simulink model "STChavelsan"  (R2015b)
settings: Solver=VariableStepAuto  StartTime=0.0  StopTime=10.0  RelTol=1e-3
settings Model: Creator=hyarkin  LastModifiedBy=hyarkin

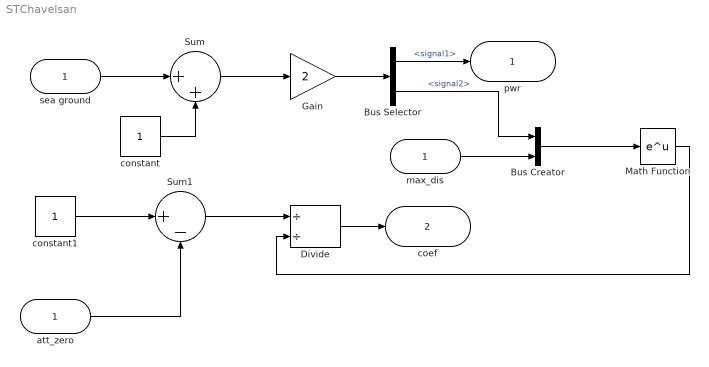
== system STChavelsan ==
  sea ground : Inport
  Bus Creator : BusCreator  Inputs=2
  Bus Selector : BusSelector  OutputSignals=signal1,signal2
  Divide : Product  Inputs=//
  Gain : Gain  Gain=2
  Math Function : Math  SaturateOnIntegerOverflow=on
  Sum : Sum  Inputs=|++
  Sum1 : Sum  Inputs=|+-
  att_zero : InportShadow
  constant : Constant  VectorParams1D=off  SampleTime=-1
  constant1 : Constant  VectorParams1D=off  SampleTime=-1
  max_dis : InportShadow
  pwr : Outport
  coef : Outport  Port=2
  wires:
  sea ground/1 -> Sum/1
  constant/1 -> Sum/2
  Sum/1 -> Gain/1
  constant1/1 -> Sum1/1
  att_zero/1 -> Sum1/2
  Gain/1 -> Bus Selector/1
  Bus Selector/1 -> pwr/1  "<signal1>"
  Bus Selector/2 -> Bus Creator/1  "<signal2>"
  max_dis/1 -> Bus Creator/2
  Bus Creator/1 -> Math Function/1
  Sum1/1 -> Divide/1
  Math Function/1 -> Divide/2
  Divide/1 -> coef/1
